simulink model "model"  (R2015a)
settings: Solver=ode3  StartTime=0.0  StopTime=2  FixedStep=dt  RelTol=1e-3
InitFcn:
  | init_sim
values from neighbouring files (symbols this model uses):
  dt = 1/100000    (= 1e-05)    [init_sim.m]
  fs = 100    [init_sim.m]
  M1 = 350    [init_sim.m]
  M2 = 3.3    [init_sim.m]
libraries: simulink x2
settings Model: Creator=Simon  LastModifiedBy=Simon

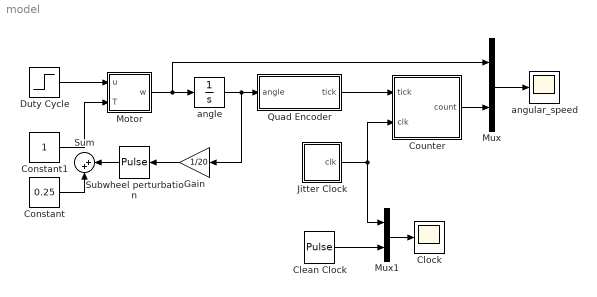
== system model ==
  Clean Clock : DiscretePulseGenerator  PulseType=Time based  Period=1/fs  PulseWidth=50
  Clock : Scope
      settings: YMin=0.9825  YMax=1.015
  Constant : Constant  Value=0.25
  Constant1 : Constant
  Counter : Subsystem
  Duty Cycle : Step  Time=0  After=.4  SampleTime=0
  Gain : Gain  Gain=1/20
  Jitter Clock : Subsystem
  Motor : Subsystem
  Mux : Mux  Inputs=2
  Mux1 : Mux  Inputs=2
  Quad Encoder : Subsystem
  Subwheel perturbation : DiscretePulseGenerator  PulseType=Time based  TimeSource=Use external signal  Amplitude=0.5  Period=1/fs  PulseWidth=5
  Sum : Sum  Inputs=|++
  angle : Integrator
  angular_speed : Scope
      settings: YMin=41.85  YMax=42.8
  wires:
  Duty Cycle/1 -> Motor/1(u)
  Mux/1 -> angular_speed/1
  Motor/1(w) -> Mux/1, angle/1
  Mux1/1 -> Clock/1
  Clean Clock/1 -> Mux1/2
  Jitter Clock/1(clk) -> Counter/2(clk), Mux1/1
  Counter/1(count) -> Mux/2
  angle/1 -> Gain/1, Quad Encoder/1(angle)
  Quad Encoder/1(tick) -> Counter/1(tick)
  Subwheel perturbation/1 -> Sum/2
  Constant/1 -> Sum/1
  Gain/1 -> Subwheel perturbation/1
  Constant1/1 -> Motor/2(T)

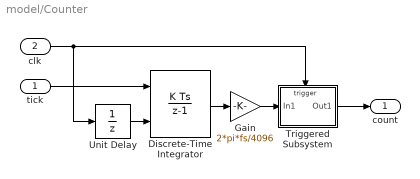
== system model/Counter ==
  tick : Inport
  clk : Inport  Port=2
  Discrete-Time Integrator : DiscreteIntegrator  gainval=1/dt  ExternalReset=rising  InitialConditionSetting=State (most efficient)  SampleTime=dt
  Gain : Gain  Gain=2*pi*fs/4096
  Triggered Subsystem : Subsystem  TreatAsAtomicUnit=on
  Unit Delay : UnitDelay  SampleTime=-1
  count : Outport
  wires:
  clk/1 -> Unit Delay/1, Triggered Subsystem/Trigger
  Unit Delay/1 -> Discrete-Time Integrator/2
  Discrete-Time Integrator/1 -> Gain/1
  Triggered Subsystem/1(Out1) -> count/1
  tick/1 -> Discrete-Time Integrator/1
  Gain/1 -> Triggered Subsystem/1(In1)

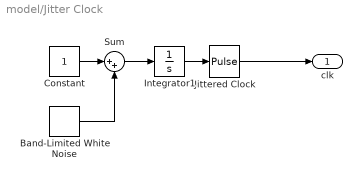
== system model/Jitter Clock ==
  Band-Limited White Noise : simulink/Sources/Band-Limited White Noise  Cov=[0.0000001]  Ts=dt  seed=[23341]
  Constant : Constant
  Integrator1 : Integrator
  Jittered Clock : DiscretePulseGenerator  PulseType=Time based  TimeSource=Use external signal  Period=1/fs  PulseWidth=50
  Sum : Sum  Inputs=|++
  clk : Outport
  wires:
  Sum/1 -> Integrator1/1
  Constant/1 -> Sum/1
  Jittered Clock/1 -> clk/1
  Band-Limited White Noise/1 -> Sum/2
  Integrator1/1 -> Jittered Clock/1

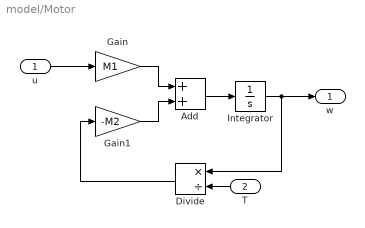
== system model/Motor ==
  u : Inport
  T : Inport  Port=2
  Add : Sum
  Divide : Product  Inputs=*/
  Gain : Gain  Gain=M1
  Gain1 : Gain  Gain=-M2
  Integrator : Integrator
  w : Outport
  wires:
  u/1 -> Gain/1
  Gain/1 -> Add/1
  Gain1/1 -> Add/2
  Add/1 -> Integrator/1
  Integrator/1 -> Divide/1, w/1
  Divide/1 -> Gain1/1
  T/1 -> Divide/2

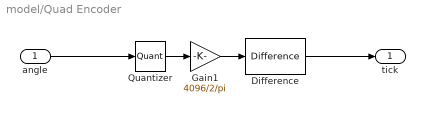
== system model/Quad Encoder ==
  angle : Inport
  Difference : simulink/Discrete/Difference  ICPrevInput=0.0  InputProcessing=Inherited  OutMin=[]  OutMax=[]  OutDataType=fixdt(1, 16)  OutScaling=2^-10  DoSatur=off
  Gain1 : Gain  Gain=4096/2/pi
  Quantizer : Quantizer  QuantizationInterval=2*pi/4096
  tick : Outport
  wires:
  Gain1/1 -> Difference/1
  Difference/1 -> tick/1
  angle/1 -> Quantizer/1
  Quantizer/1 -> Gain1/1

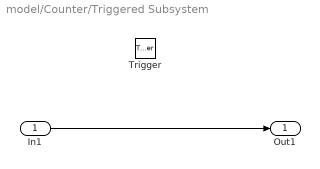
== system model/Counter/Triggered Subsystem ==
  In1 : Inport
  Trigger : TriggerPort
  Out1 : Outport
  wires:
  In1/1 -> Out1/1
